simulink model "gepnoi"  (R2018a)
settings: Solver=VariableStepAuto  StartTime=0.0  StopTime=3.0  RelTol=1e-3
InitFcn:
  | UaN = 400; IaN = 62; PN = 22e3;
  | La = 5.2e-3; Ra = 0.32;
  | TN = 67.8; nN = 3100; J = 0.05;
  | UfN = 310; IfN = 1.8;
  | eta = 0.873;
  | % Tinh toan tham so chua biet
  | KE = (UaN - Ra*IaN)*9.55/nN ;
  | KT = KE ;
  | Laf = KE/IfN ;
  | Rf = UfN/IfN ;
  | Lf = Laf ;
  | fL=200;
  | 
  | zeta=1/sqrt(2);
  | Tfv=0.001;
  | Tsp=0.05;
  | %---------------------------------------------
  | Td=1/(fL) ;
  | Tfi=1/(5*fL) ;
  | Te=Td+Tfi ;
  | Ta=La/Ra ;
  | wn=1/(2*Te*zeta) ;
  | Kp=(Ra*Ta*wn)/(2*zeta) ;
  | Ti=Ta ;
  | Ki=Kp/Ti ;
  | %----------------------------------
  | Teq=(2*zeta)/wn+Tfv ;
  | Tmech=J/KE ;
  | Tiv=4*Teq ;
  | Kpv=Tmech/(2*Teq) ;
  | Kiv=Kpv/Tiv;
undefined symbols (not defined in the file): D1, lagging, pulse
libraries: powerlib x16, powerlib_meascontrol x2
settings Model: Creator=Admin  LastModifiedBy=Admin

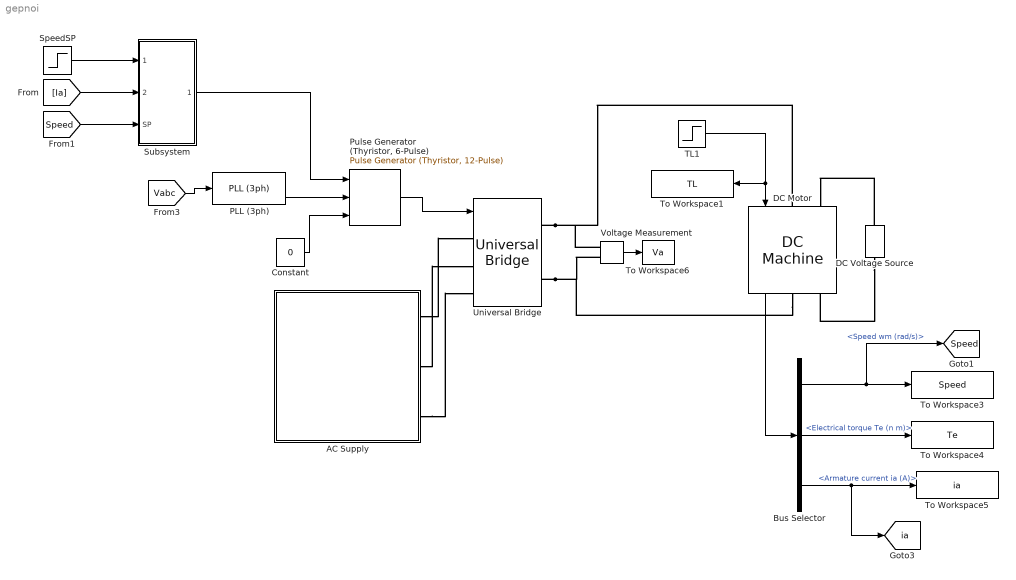
== system gepnoi ==
  AC Supply : Subsystem
  Bus Selector : BusSelector  OutputSignals=Speed wm (rad/s),Electrical torque Te (n m),Armature current ia (A)
  Constant : Constant  Value=0
  DC Motor : powerlib/Machines/DC Machine  PresetModel=No  MechanicalLoad=Torque TL  FieldType=Wound  ShowDetailedParameters=on  MeasurementBus=off  RLa="[ Ra  La]"  RLf="[ Rf  Laf/2]"  Laf=Laf  MachineConstant=Torque constant (N.m/A)  Ke=1.8  Kt=1.8  J=1  Bm=0  Tf=0  w0=0  Ifinit=1.8  TsPowergui=0  TsBlock=-1
  DC Voltage Source : powerlib/Electrical Sources/DC Voltage Source  Amplitude=UfN  Measurements=None
  PLL (3ph) : powerlib_meascontrol/PLL/PLL (3ph)  Fmin=50  Par_Init=[0, 60]  ParK=[180, 3200, 1]  TcD=1e-4  MaxRateChangeFreq=12  FilterCutOffFreq=25  Ts=0  AGC=on
  "Pulse Generator (Thyristor, 6-Pulse)" : powerlib_meascontrol/Pulse & Signal Generators/Pulse Generator (Thyristor, 12-Pulse)  GenType=6-pulse  Delta=D1 (lagging)  pwidth=60  Double_Pulse=on  Ts=0
      settings: SourceProductBaseCode=PS
  SpeedSP : Step  SampleTime=0
  Subsystem : Subsystem
  TL1 : Step  Time=0  After=TN  SampleTime=0
  To Workspace1 : ToWorkspace  VariableName=TL  SaveFormat=Structure With Time  SampleTime=1e-6
  To Workspace3 : ToWorkspace  VariableName=Speed  SaveFormat=Structure With Time  SampleTime=-1
  To Workspace4 : ToWorkspace  VariableName=Te  SaveFormat=Structure With Time  SampleTime=-1
  To Workspace5 : ToWorkspace  VariableName=ia  SaveFormat=Structure With Time  SampleTime=-1
  To Workspace6 : ToWorkspace  VariableName=Va  SaveFormat=Structure With Time  SampleTime=-1
  Universal Bridge : powerlib/Power Electronics/Universal Bridge  Arms=3  SnubberResistance=1e5  SnubberCapacitance=inf  Device=Thyristors  Ron=1e-3  Lon=0  ForwardVoltages="[  0  0  ]"  ForwardVoltage=0  GTOparameters=[ 10e-6 , 20e-6 ]  IGBTparameters=[ 1e-6 , 2e-6 ]  Measurements=None  Measurements_2=None  converterType=Rectifier
  Voltage Measurement : powerlib/Measurements/Voltage Measurement  PhasorSimulation=off  OutputType=Complex  PSBequivalent=0
  tag scope: Speed=global, ia=global
  wires:
  PLL (3ph)/2 -> "Pulse Generator (Thyristor, 6-Pulse)"/2
  Voltage Measurement/1 -> To Workspace6/1
  [Vabc] -> PLL (3ph)/1
  Constant/1 -> "Pulse Generator (Thyristor, 6-Pulse)"/3
  Bus Selector/2 -> To Workspace4/1  "<Electrical torque Te (n m)>"
  Bus Selector/3 -> [ia], To Workspace5/1  "<Armature current ia (A)>"
  Bus Selector/1 -> [Speed], To Workspace3/1  "<Speed wm (rad/s)>"
  DC Motor/1 -> Bus Selector/1
  TL1/1 -> DC Motor/1, To Workspace1/1
  "Pulse Generator (Thyristor, 6-Pulse)"/1 -> Universal Bridge/1
  Subsystem/1("alpha ") -> "Pulse Generator (Thyristor, 6-Pulse)"/1
  SpeedSP/1 -> Subsystem/1(Curent FB)
  [Ia] -> Subsystem/2(Speed FB)
  [Speed] -> Subsystem/3(SP)
  connections:
  Universal Bridge/RConn2 -- DC Motor/RConn1 -- Voltage Measurement/LConn2
  Universal Bridge/RConn1 -- Voltage Measurement/LConn1 -- DC Motor/LConn1
  AC Supply/LConn2 -- Universal Bridge/LConn2
  DC Voltage Source/LConn1 -- DC Motor/RConn2
  AC Supply/LConn3 -- Universal Bridge/LConn3
  AC Supply/LConn1 -- Universal Bridge/LConn1
  DC Voltage Source/RConn1 -- DC Motor/LConn2

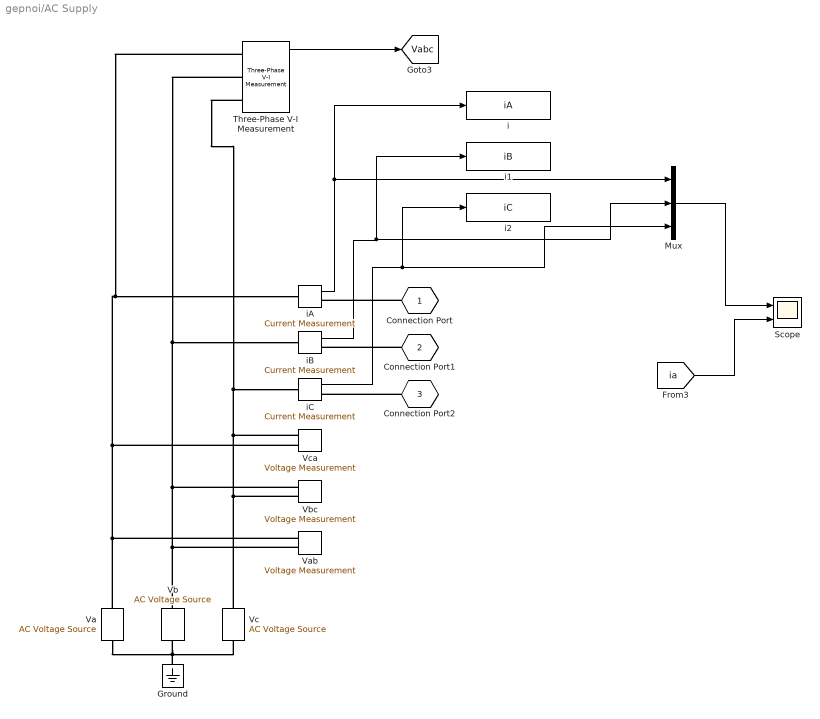
== system gepnoi/AC Supply ==
  Ground : powerlib/Elements/Ground  LConnTagsString=a
  Mux : Mux  Inputs=3
  Scope : Scope  NumInputPorts=2
  Three-Phase V-I Measurement : powerlib/Measurements/Three-Phase V-I Measurement  VoltageMeasurement=phase-to-ground  SetLabelV=off  LabelV=Vabc  Vpu=off  VpuLL=off  CurrentMeasurement=yes  SetLabelI=off  LabelI=Iabc  Ipu=off  Pbase=100e6  Vbase=500e3  OutputType=Complex  PhasorSimulation=off  PSBequivalent=0
  Va : powerlib/Electrical Sources/AC Voltage Source  Amplitude=220*sqrt(2)  Phase=0  Frequency=50  SampleTime=0  Measurements=None  BusType=swing  Pref=10e3  Qref=0  Qmin=-inf  Qmax=+inf
  Vab : powerlib/Measurements/Voltage Measurement  PhasorSimulation=off  OutputType=Complex  PSBequivalent=0
  Vb : powerlib/Electrical Sources/AC Voltage Source  Amplitude=220*sqrt(2)  Phase=-120  Frequency=50  SampleTime=0  Measurements=None  BusType=swing  Pref=10e3  Qref=0  Qmin=-inf  Qmax=+inf
  Vbc : powerlib/Measurements/Voltage Measurement  PhasorSimulation=off  OutputType=Complex  PSBequivalent=0
  Vc : powerlib/Electrical Sources/AC Voltage Source  Amplitude=220*sqrt(2)  Phase=120  Frequency=50  SampleTime=0  Measurements=None  BusType=swing  Pref=10e3  Qref=0  Qmin=-inf  Qmax=+inf
  Vca : powerlib/Measurements/Voltage Measurement  PhasorSimulation=off  OutputType=Complex  PSBequivalent=0
  i : ToWorkspace  VariableName=iA  SaveFormat=Structure With Time  SampleTime=-1
  i1 : ToWorkspace  VariableName=iB  SaveFormat=Structure With Time  SampleTime=-1
  i2 : ToWorkspace  VariableName=iC  SaveFormat=Structure With Time  SampleTime=-1
  iA : powerlib/Measurements/Current Measurement  PhasorSimulation=off  OutputType=Complex  PSBequivalent=0
  iB : powerlib/Measurements/Current Measurement  PhasorSimulation=off  OutputType=Complex  PSBequivalent=0
  iC : powerlib/Measurements/Current Measurement  PhasorSimulation=off  OutputType=Complex  PSBequivalent=0
  Connection Port : PMIOPort  Tag=PMCPort  Side=Left
  Connection Port1 : PMIOPort  Tag=PMCPort  Port=2  Side=Left
  Connection Port2 : PMIOPort  Tag=PMCPort  Port=3  Side=Left
  tag scope: Vabc=global
  wires:
  iA/1 -> Mux/1, i/1
  iB/1 -> Mux/2, i1/1
  Mux/1 -> Scope/1
  iC/1 -> Mux/3, i2/1
  Three-Phase V-I Measurement/1 -> [Vabc]
  [ia] -> Scope/2
  connections:
  Vbc/LConn2 -- Vc/RConn1 -- Three-Phase V-I Measurement/LConn3 -- iC/LConn1 -- Vca/LConn1
  Vab/LConn2 -- Vb/RConn1 -- Three-Phase V-I Measurement/LConn2 -- iB/LConn1 -- Vbc/LConn1
  Ground/LConn1 -- Va/LConn1 -- Vc/LConn1 -- Vb/LConn1
  Va/RConn1 -- Three-Phase V-I Measurement/LConn1 -- iA/LConn1 -- Vca/LConn2 -- Vab/LConn1
  Connection Port/RConn1 -- iA/RConn1
  Connection Port1/RConn1 -- iB/RConn1
  Connection Port2/RConn1 -- iC/RConn1

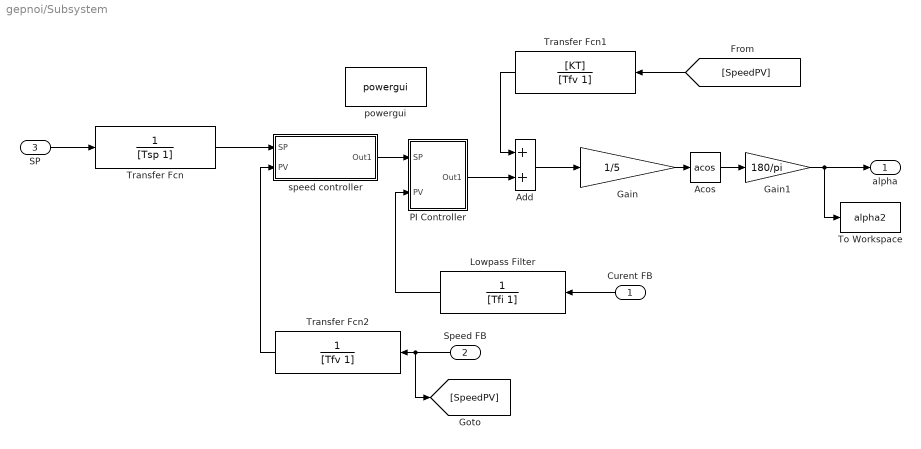
== system gepnoi/Subsystem ==
  Curent FB : Inport
  Speed FB : Inport  Port=2
  SP : Inport  Port=3
  Acos : Trigonometry  Operator=acos
  Add : Sum
  Gain : Gain  Gain=1/5
  Gain1 : Gain  Gain=180/pi
  Lowpass Filter : TransferFcn  Denominator=[Tfi 1]
  PI Controller : Subsystem
  To Workspace : ToWorkspace  VariableName=alpha2  SaveFormat=Structure With Time  SampleTime=1e-6
  Transfer Fcn : TransferFcn  Denominator=[Tsp 1]
  Transfer Fcn1 : TransferFcn  Numerator=[KT]  Denominator=[Tfv 1]
  Transfer Fcn2 : TransferFcn  Denominator=[Tfv 1]
  powergui : powerlib/powergui  Priority=1  SimulationMode=Continuous  SampleTime=50e-6  frequency=60  Iterations=50  frequencyindice=0  Pbase=100e6  ErrMax=1e-4  UnitsV=kV  UnitsW=MW  buscounter=0  FunctionMessages=off  echomessages=off  EnableUseOfTLC=off  CurrentSourceSwitches=off  DisableSnubberDevices=off  DisableRonSwitches=off  DisableVfSwitches=off  DisplayEquations=off  SolverType=Tustin/Backward Euler (TBE)  Interpol=off  ExternalGateDelay=off  methode=off  Ts=100  x0status=blocks  SPID=on  SwTol=0  HookPort=off  RestoreLinks=warning  ResistiveCurrentMeasurement=off  Frange=[0:2:500]  Ylog=off  Xlog=on  ShowGrid=off  save=off  variable=ZData  structure=0  ZoomFFT=off  StartTime=0.0  cycles=1  DisplayStyle=1  fundamental=60  FreqAxis=off  MaxFrequency=1000  frequencyindicesteady=1  RmsSteady=1  display=off
  "speed controller " : Subsystem
  "alpha " : Outport
  wires:
  Transfer Fcn/1 -> "speed controller "/1("SP ")
  PI Controller/1(Out1) -> Add/2
  [SpeedPV] -> Transfer Fcn1/1
  Transfer Fcn2/1 -> "speed controller "/2("PV ")
  Add/1 -> Gain/1
  Curent FB/1 -> Lowpass Filter/1
  Lowpass Filter/1 -> PI Controller/2(PV)
  Gain1/1 -> "alpha "/1, To Workspace/1
  Acos/1 -> Gain1/1
  Transfer Fcn1/1 -> Add/1
  "speed controller "/1(Out1) -> PI Controller/1("SP ")
  Gain/1 -> Acos/1
  Speed FB/1 -> [SpeedPV], Transfer Fcn2/1
  SP/1 -> Transfer Fcn/1

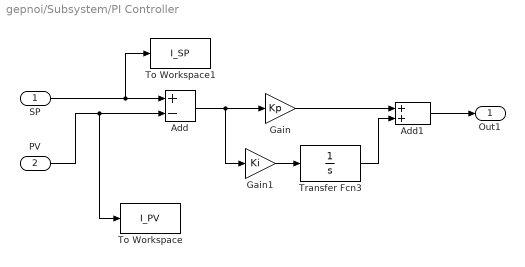
== system gepnoi/Subsystem/PI Controller ==
  "SP " : Inport
  PV : Inport  Port=2
  Add : Sum  Inputs=+-
  Add1 : Sum
  Gain : Gain  Gain=Kp
  Gain1 : Gain  Gain=Ki
  To Workspace : ToWorkspace  VariableName=I_PV  SaveFormat=Structure With Time  SampleTime=1e-6
  To Workspace1 : ToWorkspace  VariableName=I_SP  SaveFormat=Structure With Time  SampleTime=1e-6
  Transfer Fcn3 : TransferFcn  Denominator=[1 0]
  Out1 : Outport
  wires:
  Add1/1 -> Out1/1
  Transfer Fcn3/1 -> Add1/2
  Add/1 -> Gain1/1, Gain/1
  Gain/1 -> Add1/1
  Gain1/1 -> Transfer Fcn3/1
  "SP "/1 -> To Workspace1/1, Add/1
  PV/1 -> To Workspace/1, Add/2

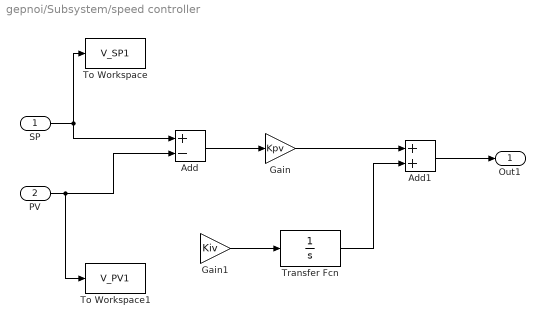
== system gepnoi/Subsystem/speed controller  ==
  "SP " : Inport
  "PV " : Inport  Port=2
  Add : Sum  Inputs=+-
  Add1 : Sum
  Gain : Gain  Gain=Kpv
  Gain1 : Gain  Gain=Kiv
  To Workspace : ToWorkspace  VariableName=V_SP1  SaveFormat=Timeseries  SampleTime=-1
  To Workspace1 : ToWorkspace  VariableName=V_PV1  SaveFormat=Timeseries  SampleTime=-1
  Transfer Fcn : TransferFcn  Denominator=[1 0]
  Out1 : Outport
  wires:
  Gain1/1 -> Transfer Fcn/1
  Gain/1 -> Add1/1
  Transfer Fcn/1 -> Add1/2
  Add/1 -> Gain/1
  Add1/1 -> Out1/1
  "SP "/1 -> Add/1, To Workspace/1
  "PV "/1 -> To Workspace1/1, Add/2
